simulink model "Complete_Model"  (R2014b)
settings: Solver=ode45  StartTime=0.0  StopTime=10.0  RelTol=1e-3
values from neighbouring files (symbols this model uses):
  C1 = (eff*K_m*K_g)/(R_a*J_eq)    (= 66.3942391304)    [Parameters.m]
  C2 = (B_eq/J_eq)+((eff*K_m*K_m*K_g*K_g)/(R_a*J_eq))    (= 37.3861974239)    [Parameters.m]
  K_d = 0.6987    [Parameters.m]
  K_d_x = 0.4985    [Parameters.m]
  K_p = 41.292    [Parameters.m]
  K_p_x = 0.87    [Parameters.m]
  L = 0.1675    [Parameters.m]
  r = 0.0254    [Parameters.m]
settings Model: Creator=USER PC  LastModifiedBy=USER PC

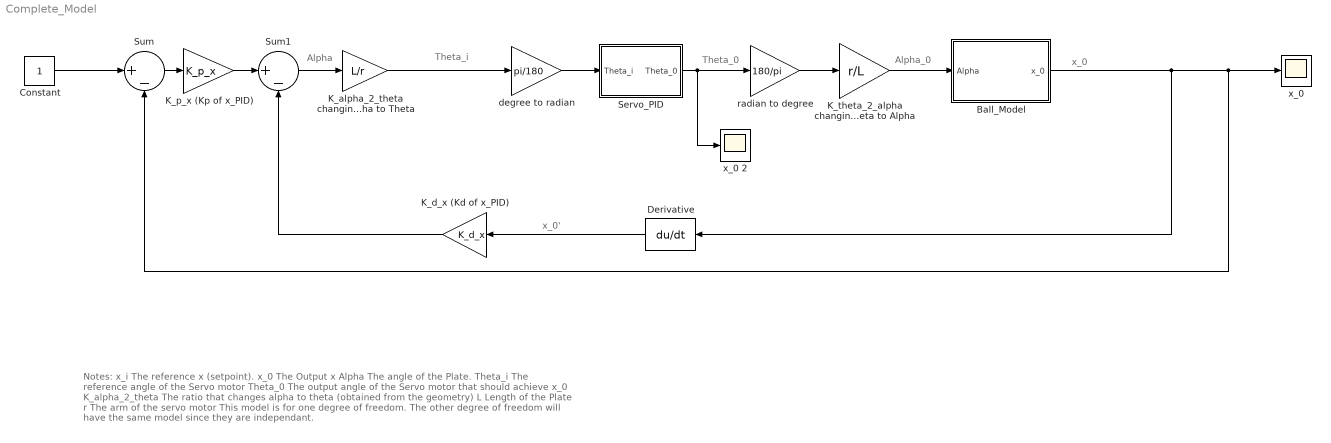
== system Complete_Model ==
  note: Notes:
      |
      | x_i The reference x (setpoint).
      | x_0 The Output x
      | Alpha The angle of the Plate.
      | Theta_i The reference angle of the Servo motor
      | Theta_0 The output angle of the Servo motor that should achieve x_0
      | K_alpha_2_theta The ratio that changes alpha to theta (obtained from the geometry)
      | L Length of the Plate
      | r The arm of the servo motor
      |
      | This model is for one degree of freedom. The other degree of freedom will have the same model since they are independant.
  note: x_0'
  note: x_0
  note: Alpha_0
  note: Theta_0
  note: Theta_i
  note: Alpha
  Ball_Model : Subsystem
  Constant : Constant
  Derivative : Derivative
  K_alpha_2_theta changing Alpha to Theta : Gain  Gain=L/r
  K_d_x (Kd of x_PID) : Gain  Gain=K_d_x
  "K_p_x (Kp of x_PID) " : Gain  Gain=K_p_x
  K_theta_2_alpha changing Theta to Alpha : Gain  Gain=r/L
  Servo_PID : Subsystem
  Sum : Sum  Inputs=|+-
  Sum1 : Sum  Inputs=|+-
  degree to radian : Gain  Gain=pi/180
  radian to degree : Gain  Gain=180/pi
  "x_0 " : Scope
  x_0 2 : Scope
      settings: SaveName=ScopeData2
  wires:
  Sum/1 -> "K_p_x (Kp of x_PID) "/1
  "K_p_x (Kp of x_PID) "/1 -> Sum1/1
  K_d_x (Kd of x_PID)/1 -> Sum1/2
  Sum1/1 -> K_alpha_2_theta changing Alpha to Theta/1
  K_alpha_2_theta changing Alpha to Theta/1 -> degree to radian/1
  K_theta_2_alpha changing Theta to Alpha/1 -> Ball_Model/1(Alpha)
  Derivative/1 -> K_d_x (Kd of x_PID)/1
  radian to degree/1 -> K_theta_2_alpha changing Theta to Alpha/1
  degree to radian/1 -> Servo_PID/1(Theta_i)
  Constant/1 -> Sum/1
  Ball_Model/1("x_0 ") -> Derivative/1, Sum/2, "x_0 "/1
  Servo_PID/1(Theta_0) -> x_0 2/1, radian to degree/1

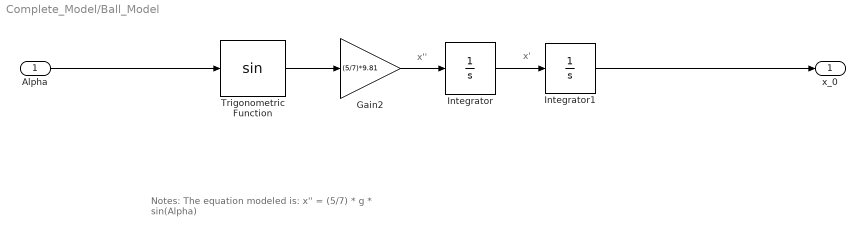
== system Complete_Model/Ball_Model ==
  note: Notes:
      |
      | The equation modeled is:
      |
      | x'' = (5/7) * g * sin(Alpha)
  note: x'
  note: x''
  Alpha : Inport
  Gain2 : Gain  Gain=(5/7)*9.81
  Integrator : Integrator
  Integrator1 : Integrator
  Trigonometric Function : Trigonometry
  "x_0 " : Outport
  wires:
  Integrator1/1 -> "x_0 "/1
  Gain2/1 -> Integrator/1
  Integrator/1 -> Integrator1/1
  Trigonometric Function/1 -> Gain2/1
  Alpha/1 -> Trigonometric Function/1

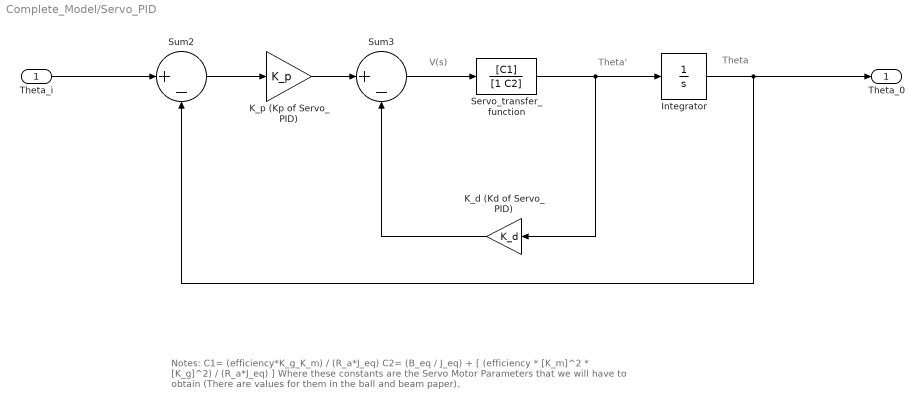
== system Complete_Model/Servo_PID ==
  note: Notes:
      |
      | C1= (efficiency*K_g_K_m) / (R_a*J_eq)
      | C2= (B_eq / J_eq) + [ (efficiency * [K_m]^2 * [K_g]^2) / (R_a*J_eq) ]
      |
      | Where these constants are the Servo Motor Parameters that we will have to obtain (There are values for them in the ball and beam paper).
  note: Theta
  note: Theta'
  note: V(s)
  Theta_i : Inport
  Integrator : Integrator
  K_d (Kd of Servo_PID) : Gain  Gain=K_d
  K_p (Kp of Servo_PID) : Gain  Gain=K_p
  "Servo_transfer_function " : TransferFcn  Numerator=[C1]  Denominator=[1 C2]
  Sum2 : Sum  Inputs=|+-
  Sum3 : Sum  Inputs=|+-
  Theta_0 : Outport
  wires:
  Theta_i/1 -> Sum2/1
  K_p (Kp of Servo_PID)/1 -> Sum3/1
  Sum2/1 -> K_p (Kp of Servo_PID)/1
  Integrator/1 -> Theta_0/1, Sum2/2
  K_d (Kd of Servo_PID)/1 -> Sum3/2
  Sum3/1 -> "Servo_transfer_function "/1
  "Servo_transfer_function "/1 -> K_d (Kd of Servo_PID)/1, Integrator/1
